simulink model "GDFLIB_FilterIIR2_BAM"  (Simulink 9.3)
settings: Solver=VariableStepAuto  StartTime=0.0  StopTime=10.0  RelTol=1e-3
settings Model: Creator=nxa18952  LastModifiedBy=nxa18952
settings DataIOCC: SaveFormat=Dataset  SignalLoggingSaveFormat=Dataset  ReturnWorkspaceOutputs=on
settings OptimizationCC: LifeSpan=auto
settings DebuggingCC: UnderspecifiedInitializationDetection=Simplified  MergeDetectMultiDrivingBlocksExec=error  FcnCallInpInsideContextMsg=error  SFUnexpectedBacktrackingDiag=error  SFNoUnconditionalDefaultTransitionDiag=error  SFExecutionAtInitializationDiag=warning  ArithmeticOperatorsInVariantConditions=error
settings HardwareCC: ProdBitPerPointer=64  ProdBitPerSizeT=64  ProdBitPerPtrDiffT=64  ProdLargestAtomicFloat=Float  ProdIntDivRoundTo=Zero  ProdEndianess=LittleEndian  ProdWordSize=64  ProdHWDeviceType=Intel->x86-64 (Windows64)
settings ModelReferenceCC: PropagateSignalLabelsOutOfModel=on
settings SFSimCC: SimUseLocalCustomCode=on
settings RTWCC: RTWUseLocalCustomCode=on
settings CodeAppCC: StateflowObjectComments=off
settings GRTTargetCC: TargetLangStandard=C99 (ISO)  CombineOutputUpdateFcns=on  GRTInterface=off
settings ConfigComp: CovMetricSettings=dwe  CovHtmlReporting=off  CovSaveCumulativeToWorkspaceVar=off  CovSaveSingleToWorkspaceVar=off  CovExternalEMLEnable=on

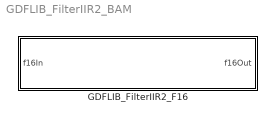
== system GDFLIB_FilterIIR2_BAM ==
  GDFLIB_FilterIIR2_F16 : Subsystem  TreatAsAtomicUnit=on  mask(GDFLIB_FilterIIR2_F16){showStates=Hide (faster execution), f16B0=0, f16B1=0, f16B2=0, f16A1=0, f16A2=0}
      mask prompts: showStates "Show internal states"; f16B0 "f16B0 (B0 coefficient of the IIR2 filter in 16-bit fixed-point fractional format)"; f16B1 "f16B1 (B1 coefficient of the IIR2 filter in 16-bit fixed-point fractional format)"; f16B2 "f16B2 (B2 coefficient of the IIR2 filter in 16-bit fixed-point fractional format)"; f16A1 "f16A1 (A1 coefficient of the IIR2 filter in 16-bit fixed-point fractional format)"; f16A2 "f16A2 (A2 coefficient of the IIR2 filter in 16-bit fixed-point fractional format)"
      mask help: Direct form I second order IIR filter in 16-bit fixed-point fractional implementation. Refer to the AMMCLIB User's Guide for further details.
      mask init:
      | if ~evalin('base','exist(''tS8'',''var'')')
      |   if (2 ~= exist('SWLIBS_Typedefs.mat','file'))
      |       error('File SWLIBS_Typedefs.mat is not on the Matlab path. Please add the AMMCLIB "bam" folder in the Matlab Search Path.');
      |   else
      |       evalin('base', 'load(''SWLIBS_Typedefs.mat'')');
      |   end
      | end
      | if showStates == 1
      |     % hidden state variables
      |     if strcmp(get_param([gcb '/f16FiltBufferX1'], 'BlockType'), 'Inport')
      |         posblk = get_param(gcb, 'Position');
      | 
      |         pos = get_param(    [gcb, '/f16FiltBufferX1'], 'Position');
      |         orient = get_param( [gcb, '/f16FiltBufferX1'], 'Orientation');
      |         delete_block(       [gcb, '/f16FiltBufferX1']);
      |         add_block('built-in/Ground', [gcb, '/f16FiltBufferX1'], 'Position', pos, 'Orientation', orient);
      | 
      |         pos = get_param(    [gcb, '/f16FiltBufferX2'], 'Position');
      |         orient = get_param( [gcb, '/f16FiltBufferX2'], 'Orientation');
      |         delete_block(       [gcb, '/f16FiltBufferX2']);
      |         add_block('built-in/Ground', [gcb, '/f16FiltBufferX2'], 'Position', pos, 'Orientation', orient);
      | 
      |         pos = get_param(    [gcb, '/f32FiltBufferY1'], 'Position');
      |         orient = get_param( [gcb, '/f32FiltBufferY1'], 'Orientation');
      |         delete_block(       [gcb, '/f32FiltBufferY1']);
      |         add_block('built-in/Ground', [gcb, '/f32FiltBufferY1'], 'Position', pos, 'Orientation', orient);
      | 
      |         pos = get_param(    [gcb, '/f32FiltBufferY2'], 'Position');
      |         orient = get_param( [gcb, '/f32FiltBufferY2'], 'Orientation');
      |         delete_block(       [gcb, '/f32FiltBufferY2']);
      |         add_block('built-in/Ground', [gcb, '/f32FiltBufferY2'], 'Position', pos, 'Orientation', orient);
      | 
      |         pos = get_param(    [gcb, '/f16B0'], 'Position');
      |         orient = get_param( [gcb, '/f16B0'], 'Orientation');
      |         delete_block(       [gcb, '/f16B0']);
      |         add_block('built-in/Ground', [gcb, '/f16B0'], 'Position', pos, 'Orientation', orient);
      | 
      |         pos = get_param(    [gcb, '/f16B1'], 'Position');
      |         orient = get_param( [gcb, '/f16B1'], 'Orientation');
      |         delete_block(       [gcb, '/f16B1']);
      |         add_block('built-in/Ground', [gcb, '/f16B1'], 'Position', pos, 'Orientation', orient);
      | 
      |         pos = get_param(    [gcb, '/f16B2'], 'Position');
      |         orient = get_param( [gcb, '/f16B2'], 'Orientation');
      |         delete_block(       [gcb, '/f16B2']);
      |         add_block('built-in/Ground', [gcb, '/f16B2'], 'Position', pos, 'Orientation', orient);
      | 
      |         pos = get_param(    [gcb, '/f16A1'], 'Position');
      |         orient = get_param( [gcb, '/f16A1'], 'Orientation');
      |         delete_block(       [gcb, '/f16A1']);
      |         add_block('built-in/Ground', [gcb, '/f16A1'], 'Position', pos, 'Orientation', orient);
      | 
      |         pos = get_param(    [gcb, '/f16A2'], 'Position');
      |         orient = get_param( [gcb, '/f16A2'], 'Orientation');
      |         delete_block(       [gcb, '/f16A2']);
      |         add_block('built-in/Ground', [gcb, '/f16A2'], 'Position', pos, 'Orientation', orient);
      | 
      | 
      |         pos = get_param(    [gcb '/FilterBufferX1_Out'], 'Position');
      |         orient = get_param( [gcb '/FilterBufferX1_Out'], 'Orientation');
      |         delete_block(       [gcb '/FilterBufferX1_Out']);
      |         add_block('built-in/Terminator', [gcb '/FilterBufferX1_Out'], 'Position', pos, 'Orientation', orient);
      | 
      |         pos = get_param(    [gcb '/FilterBufferX2_Out'], 'Position');
      |         orient = get_param( [gcb '/FilterBufferX2_Out'], 'Orientation');
      |         delete_block(       [gcb '/FilterBufferX2_Out']);
      |         add_block('built-in/Terminator', [gcb '/FilterBufferX2_Out'], 'Position', pos, 'Orientation', orient);
      | 
      |         pos = get_param(    [gcb '/FilterBufferY1_Out'], 'Position');
      |         orient = get_param( [gcb '/FilterBufferY1_Out'], 'Orientation');
      |         delete_block(       [gcb '/FilterBufferY1_Out']);
      |         add_block('built-in/Terminator', [gcb '/FilterBufferY1_Out'], 'Position', pos, 'Orientation', orient);
      | 
      |         pos = get_param(    [gcb '/FilterBufferY2_Out'], 'Position');
      |         orient = get_param( [gcb '/FilterBufferY2_Out'], 'Orientation');
      |         delete_block(       [gcb '/FilterBufferY2_Out']);
      |         add_block('built-in/Terminator', [gcb '/FilterBufferY2_Out'], 'Position', pos, 'Orientation', orient);
      | 
      | 
      |         set_param([gcb '/f16In'], 'Port', '1');
      | 
      |         set_param([gcb '/f16Out'], 'Port', '1');
      | 
      |         set_param(gcb,'MaskEnables',{'on','on','on','on','on','on'});
      | 
      |         if (posblk(4) - posblk(2)) > 50
      |           height = 50;
      |           set_param(gcb,'Position',[posblk(1), posblk(2), posblk(3), posblk(2)+height])
      |         end
      |     end
      | else
      |     % shown state variables
      |     if strcmp(get_param([gcb '/f16FiltBufferX1'], 'BlockType'), 'Ground')
      |         posblk = get_param(gcb, 'Position');
      | 
      |         pos = get_param(    [gcb, '/f16FiltBufferX1'], 'Position');
      |         orient = get_param( [gcb, '/f16FiltBufferX1'], 'Orientation');
      |         delete_block(       [gcb, '/f16FiltBufferX1']);
      |         add_block('built-in/Inport', [gcb, '/f16FiltBufferX1'], 'Position', pos, 'Orientation', orient, 'OutDataTypeStr', 'int16');
      | 
      |         pos = get_param(    [gcb, '/f16FiltBufferX2'], 'Position');
      |         orient = get_param( [gcb, '/f16FiltBufferX2'], 'Orientation');
      |         delete_block(       [gcb, '/f16FiltBufferX2']);
      |         add_block('built-in/Inport', [gcb, '/f16FiltBufferX2'], 'Position', pos, 'Orientation', orient, 'OutDataTypeStr', 'int16');
      | 
      |         pos = get_param(    [gcb, '/f32FiltBufferY1'], 'Position');
      |         orient = get_param( [gcb, '/f32FiltBufferY1'], 'Orientation');
      |         delete_block(       [gcb, '/f32FiltBufferY1']);
      |         add_block('built-in/Inport', [gcb, '/f32FiltBufferY1'], 'Position', pos, 'Orientation', orient, 'OutDataTypeStr', 'int32');
      | 
      |         pos = get_param(    [gcb, '/f32FiltBufferY2'], 'Position');
      |         orient = get_param( [gcb, '/f32FiltBufferY2'], 'Orientation');
      |         delete_block(       [gcb, '/f32FiltBufferY2']);
      |         add_block('built-in/Inport', [gcb, '/f32FiltBufferY2'], 'Position', pos, 'Orientation', orient, 'OutDataTypeStr', 'int32');
      | 
      |         pos = get_param(    [gcb, '/f16B0'], 'Position');
      |         orient = get_param( [gcb, '/f16B0'], 'Orientation');
      |         delete_block(       [gcb, '/f16B0']);
      |         add_block('built-in/Inport', [gcb, '/f16B0'], 'Position', pos, 'Orientation', orient, 'OutDataTypeStr', 'int16');
      | 
      |         pos = get_param(    [gcb, '/f16B1'], 'Position');
      |         orient = get_param( [gcb, '/f16B1'], 'Orientation');
      |         delete_block(       [gcb, '/f16B1']);
      |         add_block('built-in/Inport', [gcb, '/f16B1'], 'Position', pos, 'Orientation', orient, 'OutDataTypeStr', 'int16');
      | 
      |         pos = get_param(    [gcb, '/f16B2'], 'Position');
      |         orient = get_param( [gcb, '/f16B2'], 'Orientation');
      |         delete_block(       [gcb, '/f16B2']);
      |         add_block('built-in/Inport', [gcb, '/f16B2'], 'Position', pos, 'Orientation', orient, 'OutDataTypeStr', 'int16');
      | 
      |         pos = get_param(    [gcb, '/f16A1'], 'Position');
      |         orient = get_param( [gcb, '/f16A1'], 'Orientation');
      |         delete_block(       [gcb, '/f16A1']);
      |         add_block('built-in/Inport', [gcb, '/f16A1'], 'Position', pos, 'Orientation', orient, 'OutDataTypeStr', 'int16');
      | 
      |         pos = get_param(    [gcb, '/f16A2'], 'Position');
      |         orient = get_param( [gcb, '/f16A2'], 'Orientation');
      |         delete_block(       [gcb, '/f16A2']);
      |         add_block('built-in/Inport', [gcb, '/f16A2'], 'Position', pos, 'Orientation', orient, 'OutDataTypeStr', 'int16');
      | 
      | 
      |         pos = get_param(    [gcb '/FilterBufferX1_Out'], 'Position');
      |         orient = get_param( [gcb '/FilterBufferX1_Out'], 'Orientation');
      |         delete_block(       [gcb '/FilterBufferX1_Out']);
      |         add_block('built-in/Outport', [gcb '/FilterBufferX1_Out'], 'Position', pos, 'Orientation', orient);
      | 
      |         pos = get_param(    [gcb '/FilterBufferX2_Out'], 'Position');
      |         orient = get_param( [gcb '/FilterBufferX2_Out'], 'Orientation');
      |         delete_block(       [gcb '/FilterBufferX2_Out']);
      |         add_block('built-in/Outport', [gcb '/FilterBufferX2_Out'], 'Position', pos, 'Orientation', orient);
      | 
      |         pos = get_param(    [gcb '/FilterBufferY1_Out'], 'Position');
      |         orient = get_param( [gcb '/FilterBufferY1_Out'], 'Orientation');
      |         delete_block(       [gcb '/FilterBufferY1_Out']);
      |         add_block('built-in/Outport', [gcb '/FilterBufferY1_Out'], 'Position', pos, 'Orientation', orient);
      | 
      |         pos = get_param(    [gcb '/FilterBufferY2_Out'], 'Position');
      |         orient = get_param( [gcb '/FilterBufferY2_Out'], 'Orientation');
      |         delete_block(       [gcb '/FilterBufferY2_Out']);
      |         add_block('built-in/Outport', [gcb '/FilterBufferY2_Out'], 'Position', pos, 'Orientation', orient);
      | 
      | 
      |         set_param([gcb '/f16In'], 'Port', '1');
      |         set_param([gcb '/f16FiltBufferX1'], 'Port', '2');
      |         set_param([gcb '/f16FiltBufferX2'], 'Port', '3');
      |         set_param([gcb '/f32FiltBufferY1'], 'Port', '4');
      |         set_param([gcb '/f32FiltBufferY2'], 'Port', '5');
      |         set_param([gcb '/f16B0'], 'Port', '6');
      |         set_param([gcb '/f16B1'], 'Port', '7');
      |         set_param([gcb '/f16B2'], 'Port', '8');
      |         set_param([gcb '/f16A1'], 'Port', '9');
      |         set_param([gcb '/f16A2'], 'Port', '10');
      | 
      |         set_param([gcb '/f16Out'], 'Port', '1');
      |         set_param([gcb '/FilterBufferX1_Out'], 'Port', '2');
      |         set_param([gcb '/FilterBufferX2_Out'], 'Port', '3');
      |         set_param([gcb '/FilterBufferY1_Out'], 'Port', '4');
      |         set_param([gcb '/FilterBufferY2_Out'], 'Port', '5');
      | 
      |         set_param(gcb,'MaskEnables',{'on','off','off','off','off','off'});
      | 
      |         if (posblk(4) - posblk(2)) < 275
      |           height = 275;
      |           set_param(gcb,'Position',[posblk(1), posblk(2), posblk(3), posblk(2)+height])
      |         end
      |     end
      | end
      settings: RTWSystemCode=Inline
      mask TypeOptions showStates: Hide (faster execution) | Show (allows debugging; connect feedback loops manually)
      mask Callback showStates:
      | maskStr = get_param(gcb,'showStates');
      | if strcmp(maskStr,'Hide (faster execution)'),
      |     set_param(gcb,'MaskEnables',{'on','on','on','on','on','on'});
      | else
      |     set_param(gcb,'MaskEnables',{'on','off','off','off','off','off'});
      | end
      mask Display:
      | color('black');
      | pos = get_param(gcb, 'Position');
      | width = pos(3) - pos(1);
      | height = pos(4) - pos(2);
      | tX=width/2;
      | tY=height - 8;
      | color('black');
      | text(tX,tY, 'GDFLIB_FilterIIR2_F16', 'horizontalAlignment', 'center');
      | if showStates == 2
      |   color('red');
      |   text(tX,tY - 20, ['debugging mode' char(13) char(10) '(limited performance)'], 'horizontalAlignment', 'center');
      | end

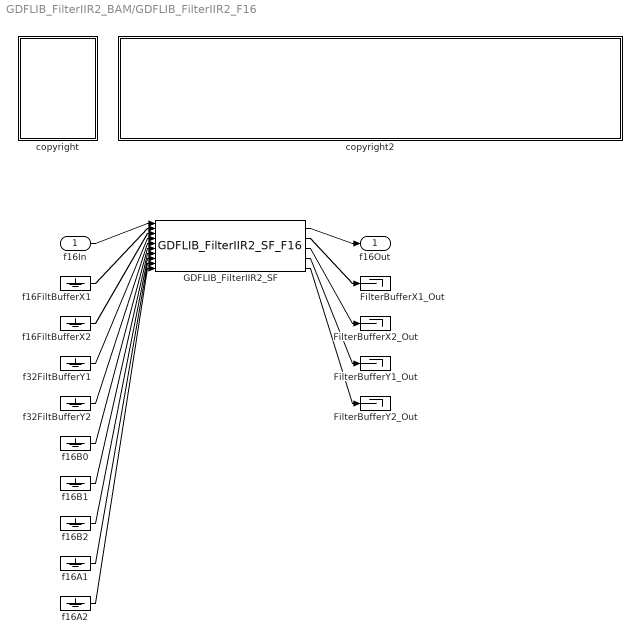
== system GDFLIB_FilterIIR2_BAM/GDFLIB_FilterIIR2_F16 ==
  f16In : Inport  OutDataTypeStr=int16
  FilterBufferX1_Out : Terminator
  FilterBufferX2_Out : Terminator
  FilterBufferY1_Out : Terminator
  FilterBufferY2_Out : Terminator
  GDFLIB_FilterIIR2_SF : S-Function  FunctionName=GDFLIB_FilterIIR2_SF_F16  Parameters=showStates,f16B0,f16B1,f16B2,f16A1,f16A2  SFunctionDeploymentMode=off  EnableBusSupport=off
  copyright : Subsystem
      mask Display: text(10,90,'FILE:');text(10,75,'DESRIPTION:');text(10,60,'COPYRIGHT:');text(10,45,'VERSION:');text(10,30,'DATE:')
  copyright2 : Subsystem
      mask Display: text(10,90,'GDFLIB_FilterIIR2_BAM_F16.mdl');text(10,75,'First order IIR filter.');text(10,60,'NXP 2020');text(10,45,'1.0');text(10,30,'18-Mar-2020');
  f16A1 : Ground
  f16A2 : Ground
  f16B0 : Ground
  f16B1 : Ground
  f16B2 : Ground
  f16FiltBufferX1 : Ground
  f16FiltBufferX2 : Ground
  f32FiltBufferY1 : Ground
  f32FiltBufferY2 : Ground
  f16Out : Outport
  wires:
  f16In/1 -> GDFLIB_FilterIIR2_SF/1
  f16FiltBufferX1/1 -> GDFLIB_FilterIIR2_SF/2
  f16FiltBufferX2/1 -> GDFLIB_FilterIIR2_SF/3
  f32FiltBufferY1/1 -> GDFLIB_FilterIIR2_SF/4
  f32FiltBufferY2/1 -> GDFLIB_FilterIIR2_SF/5
  f16B0/1 -> GDFLIB_FilterIIR2_SF/6
  f16B1/1 -> GDFLIB_FilterIIR2_SF/7
  f16B2/1 -> GDFLIB_FilterIIR2_SF/8
  f16A1/1 -> GDFLIB_FilterIIR2_SF/9
  f16A2/1 -> GDFLIB_FilterIIR2_SF/10
  GDFLIB_FilterIIR2_SF/1 -> f16Out/1
  GDFLIB_FilterIIR2_SF/2 -> FilterBufferX1_Out/1
  GDFLIB_FilterIIR2_SF/3 -> FilterBufferX2_Out/1
  GDFLIB_FilterIIR2_SF/4 -> FilterBufferY1_Out/1
  GDFLIB_FilterIIR2_SF/5 -> FilterBufferY2_Out/1

== system GDFLIB_FilterIIR2_BAM/GDFLIB_FilterIIR2_F16/copyright ==

== system GDFLIB_FilterIIR2_BAM/GDFLIB_FilterIIR2_F16/copyright2 ==
